simulink model "get_accel"  (R2018b)
settings: Solver=FixedStepAuto  StartTime=0.0  StopTime=10.0  FixedStep=0.01  RelTol=1e-3
values from neighbouring files (symbols this model uses):
  ax = polys_vals(polys_x,ts,tt,2)    [generate_trajectory.m]    (also in minJerk.m; minSnap.m)
  ay = polys_vals(polys_y,ts,tt,2)    [generate_trajectory.m]    (also in minJerk.m; minSnap.m)
  az = polys_vals(polys_z,ts,tt,2)    [generate_trajectory.m]    (also in minJerk.m; minSnap.m)
settings Model: Creator=jacky.kong  LastModifiedBy=jacky.kong

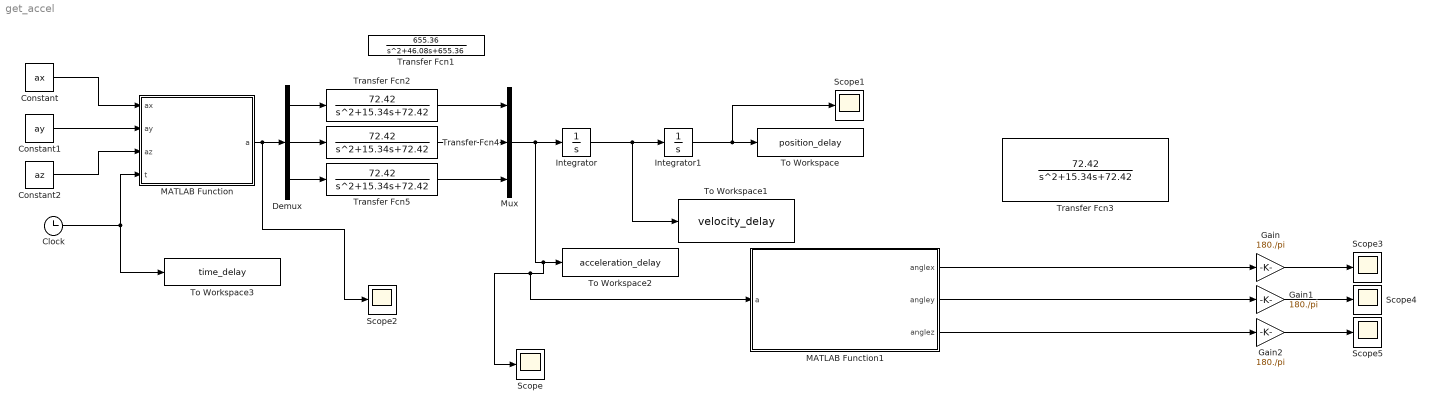
== system get_accel ==
  Clock : Clock
  Constant : Constant  Value=ax
  Constant1 : Constant  Value=ay
  Constant2 : Constant  Value=az
  Demux : Demux  Outputs=3
  Gain : Gain  Gain=180./pi
  Gain1 : Gain  Gain=180./pi
  Gain2 : Gain  Gain=180./pi
  Integrator : Integrator
  Integrator1 : Integrator
  MATLAB Function : MATLAB Function  TreatAsAtomicUnit=on
  MATLAB Function1 : MATLAB Function  TreatAsAtomicUnit=on
  Mux : Mux  Inputs=3
  Scope{,1..5} (6 alike) : Scope
  To Workspace : ToWorkspace  VariableName=position_delay  SampleTime=-1
  To Workspace1 : ToWorkspace  VariableName=velocity_delay  SampleTime=-1
  To Workspace2 : ToWorkspace  VariableName=acceleration_delay  SampleTime=-1
  To Workspace3 : ToWorkspace  VariableName=time_delay  SampleTime=-1
  Transfer Fcn1 : TransferFcn  Numerator=[655.36]  Denominator=[1 46.08 655.36]
  Transfer Fcn{2..5} (4 alike) : TransferFcn  Numerator=[72.42]  Denominator=[1 15.34 72.42]
  wires:
  Constant/1 -> MATLAB Function/1(ax)
  Constant1/1 -> MATLAB Function/2(ay)
  Constant2/1 -> MATLAB Function/3(az)
  Clock/1 -> To Workspace3/1, MATLAB Function/4(t)
  Integrator/1 -> To Workspace1/1, Integrator1/1
  Integrator1/1 -> Scope1/1, To Workspace/1
  MATLAB Function/1(a) -> Scope2/1, Demux/1
  Demux/1 -> Transfer Fcn2/1
  Mux/1 -> MATLAB Function1/1(a), Scope/1, To Workspace2/1, Integrator/1
  Transfer Fcn2/1 -> Mux/1
  Transfer Fcn4/1 -> Mux/2
  Demux/2 -> Transfer Fcn4/1
  Demux/3 -> Transfer Fcn5/1
  Transfer Fcn5/1 -> Mux/3
  Gain/1 -> Scope3/1
  Gain1/1 -> Scope4/1
  MATLAB Function1/2(angley) -> Gain1/1
  MATLAB Function1/3(anglez) -> Gain2/1
  Gain2/1 -> Scope5/1
  MATLAB Function1/1(anglex) -> Gain/1

== matlab function get_accel/MATLAB Function1 ==
  data: a input; anglex output; angley output; anglez output
function [anglex,angley,anglez] = fcn(a)

ax=a(1);
ay=a(2);
az=a(3)+9.8;
a_new = [ax ay az]';

v1 = a_new./norm(a_new);
v2 = [0 0 1]';
%转为单位向量
nv1 = v1/norm(v1);
nv2 = v2/norm(v2);
 
if norm(nv1+nv2)==0 || (norm(nv1.*nv2) == 0)
    q = [1 0 0 0]';
else
    u = cross(nv1,nv2);         
    u = u/norm(u);
    
    theta = acos(sum(nv1.*nv2))/2;
    q = [cos(theta); sin(theta)*u];
end

%由四元数构造旋转矩阵
R=[2*q(1).^2-1+2*q(2)^2  2*(q(2)*q(3)+q(1)*q(4)) 2*(q(2)*q(4)-q(1)*q(3));
    2*(q(2)*q(3)-q(1)*q(4)) 2*q(1)^2-1+2*q(3)^2 2*(q(3)*q(4)+q(1)*q(2));
    2*(q(2)*q(4)+q(1)*q(3)) 2*(q(3)*q(4)-q(1)*q(2)) 2*q(1)^2-1+2*q(4)^2];

coder.extrinsic('dcm2angle');

anglex = 0;
angley = 0;
anglez = 0;
[anglex angley anglez] = dcm2angle(R,'XYZ');

== matlab function get_accel/MATLAB Function ==
  data: ax input; a output; ay input; az input; t input
function a = get_accel(ax,ay,az,t)
max = 613
index = ceil(t./0.01)+1;
a = zeros(3,1);
if index <= 613
    a(1) = ax(index);
    a(2) = ay(index);
    a(3) = az(index);
else 
    a = [0 0 0]';
end
